simulink model "Coeff_converter_0"  (R2018b)
settings: Solver=VariableStepAuto  StartTime=0.0  StopTime=256  RelTol=1e-3
libraries: xbsIndex_r4 x38
settings Model: Creator=Dima  LastModifiedBy=Dima

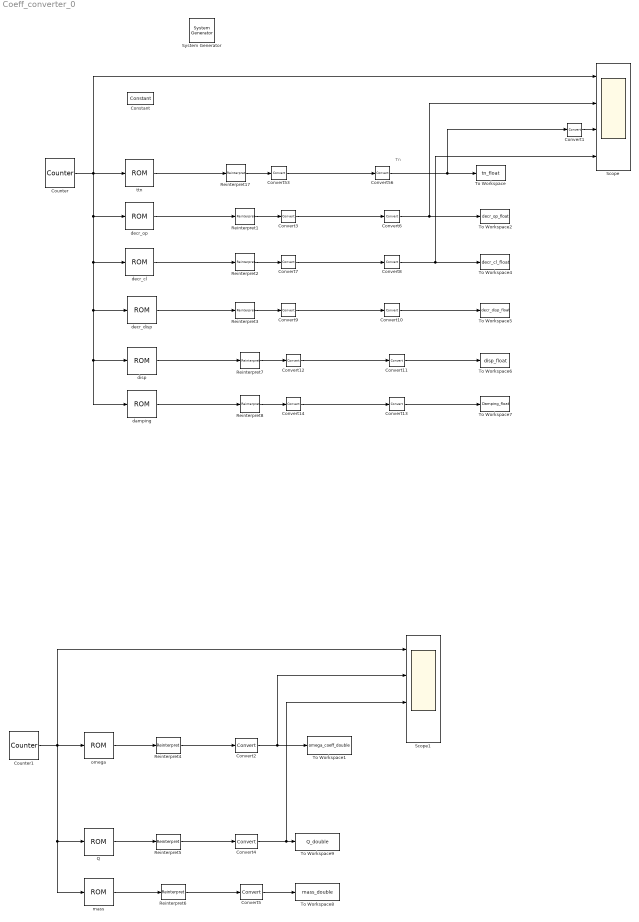
== system Coeff_converter_0 ==
  note: Tn
  " System Generator" : xbsIndex_r4/ System Generator  Tag=genX  xilinxfamily=artix7  part=xc7a35t  speed=-2  package=ftg256  synthesis_tool=Vivado  clock_wrapper=Clock Enables  directory=./netlist  proj_type=Vivado  Synth_file=Vivado Synthesis Defaults  Impl_file=Vivado Implementation Defaults  testbench=off  simulink_period=1  sysclk_period=10  dcm_input_clock_period=10  incr_netlist=off  trim_vbits=Everywhere in SubSystem  dbl_ovrd=According to Block Masks  core_generation=According to Block Masks  run_coregen=off  deprecated_control=off  eval_field=0  block_type=sysgen
  Constant : xbsIndex_r4/Constant  const=18460.73714  gui_display_data_type=Fixed-point  arith_type=Unsigned  n_bits=24  bin_pt=0  preci_type=Single  exp_width=8  frac_width=24  explicit_period=off  period=1  equ=P=C  opselect=C  inp2=PCIN>>17  opr=+  inp1=P  carry=CIN  dbl_ovrd=off  block_type=constant
  Convert{1,6,8,10..11,13,56} (7 alike) : xbsIndex_r4/Convert  gui_display_data_type=Floating-point  arith_type=Floating-point  n_bits=16  bin_pt=14  float_type=Single  exp_bits=8  fraction_bits=24  quantization=Truncate  overflow=Wrap  en=off  latency=0  pipeline=off  dbl_ovrd=off  block_type=convert
  Convert{3,7,9,12,14,53} (6 alike) : xbsIndex_r4/Convert  gui_display_data_type=Fixed-point  arith_type="Signed  (2's comp)"  n_bits=24  bin_pt=23  float_type=Single  exp_bits=8  fraction_bits=24  quantization=Truncate  overflow=Wrap  en=off  latency=0  pipeline=off  dbl_ovrd=off  block_type=convert
  Convert2 : xbsIndex_r4/Convert  gui_display_data_type=Floating-point  arith_type=Floating-point  n_bits=16  bin_pt=14  float_type=Double  exp_bits=8  fraction_bits=24  quantization=Truncate  overflow=Wrap  en=off  latency=0  pipeline=off  dbl_ovrd=off  block_type=convert
  Convert4 : xbsIndex_r4/Convert  gui_display_data_type=Floating-point  arith_type=Floating-point  n_bits=16  bin_pt=14  float_type=Double  exp_bits=8  fraction_bits=24  quantization=Truncate  overflow=Wrap  en=off  latency=0  pipeline=off  dbl_ovrd=off  block_type=convert
  Convert5 : xbsIndex_r4/Convert  gui_display_data_type=Floating-point  arith_type=Floating-point  n_bits=16  bin_pt=14  float_type=Double  exp_bits=8  fraction_bits=24  quantization=Truncate  overflow=Wrap  en=off  latency=0  pipeline=off  dbl_ovrd=off  block_type=convert
  Counter : xbsIndex_r4/Counter  cnt_type=Count Limited  cnt_to=87  operation=Up  start_count=0  cnt_by_val=1  arith_type=Unsigned  n_bits=7  bin_pt=0  load_pin=off  rst=off  en=off  explicit_period=on  period=1  use_behavioral_HDL=off  implementation=Fabric  dbl_ovrd=off  block_type=counter
  Counter1 : xbsIndex_r4/Counter  cnt_type=Free Running  cnt_to=87  operation=Up  start_count=0  cnt_by_val=1  arith_type=Unsigned  n_bits=8  bin_pt=0  load_pin=off  rst=off  en=off  explicit_period=on  period=1  use_behavioral_HDL=off  implementation=Fabric  dbl_ovrd=off  block_type=counter
  Q : xbsIndex_r4/ROM  depth=256  initVector=omega_coef  distributed_mem=Block RAM  rst=off  init_reg=0  en=off  latency=1  gui_display_data_type=Fixed-point  arith_type=Unsigned  n_bits=32  bin_pt=0  preci_type=Single  exp_width=8  frac_width=24  optimize=Area  use_rpm=on  dbl_ovrd=off  block_type=sprom
  Reinterpret{1..3,7..8,17} (6 alike) : xbsIndex_r4/Reinterpret  force_arith_type=off  arith_type="Signed  (2's comp)"  force_bin_pt=on  bin_pt=24  block_type=cast
      settings: block_version=VER_STRING_GOES_HERE
  Reinterpret4 : xbsIndex_r4/Reinterpret  force_arith_type=on  arith_type="Signed  (2's comp)"  force_bin_pt=on  bin_pt=31  block_type=reinterpret
  Reinterpret5 : xbsIndex_r4/Reinterpret  force_arith_type=on  arith_type="Signed  (2's comp)"  force_bin_pt=on  bin_pt=31  block_type=reinterpret
  Reinterpret6 : xbsIndex_r4/Reinterpret  force_arith_type=on  arith_type="Signed  (2's comp)"  force_bin_pt=on  bin_pt=31  block_type=reinterpret
  Scope : Scope  NumInputPorts=4
  Scope1 : Scope  NumInputPorts=4
  To Workspace : ToWorkspace  VariableName=tn_float  SampleTime=-1
  To Workspace1 : ToWorkspace  VariableName=omega_coeff_double  SampleTime=-1
  To Workspace2 : ToWorkspace  VariableName=decr_op_float  SampleTime=-1
  To Workspace4 : ToWorkspace  VariableName=decr_cl_float  SampleTime=-1
  To Workspace5 : ToWorkspace  VariableName=decr_disp_float  SampleTime=-1
  To Workspace6 : ToWorkspace  VariableName=disp_float  SampleTime=-1
  To Workspace7 : ToWorkspace  VariableName=Damping_float  SampleTime=-1
  To Workspace8 : ToWorkspace  VariableName=mass_double  SampleTime=-1
  To Workspace9 : ToWorkspace  VariableName=Q_double  SampleTime=-1
  damping : xbsIndex_r4/ROM  depth=88  initVector=damping  distributed_mem=Block RAM  rst=off  init_reg=0  en=off  latency=1  gui_display_data_type=Fixed-point  arith_type=Unsigned  n_bits=24  bin_pt=0  preci_type=Single  exp_width=8  frac_width=24  optimize=Area  use_rpm=on  dbl_ovrd=off  block_type=sprom
  decr_cl : xbsIndex_r4/ROM  depth=88  initVector=decr_cl  distributed_mem=Block RAM  rst=off  init_reg=0  en=off  latency=1  gui_display_data_type=Fixed-point  arith_type=Unsigned  n_bits=24  bin_pt=0  preci_type=Single  exp_width=8  frac_width=24  optimize=Area  use_rpm=on  dbl_ovrd=off  block_type=sprom
  decr_disp : xbsIndex_r4/ROM  depth=88  initVector=decr_disp  distributed_mem=Block RAM  rst=off  init_reg=0  en=off  latency=1  gui_display_data_type=Fixed-point  arith_type=Unsigned  n_bits=24  bin_pt=0  preci_type=Single  exp_width=8  frac_width=24  optimize=Area  use_rpm=on  dbl_ovrd=off  block_type=sprom
  decr_op : xbsIndex_r4/ROM  depth=88  initVector=decr_op  distributed_mem=Block RAM  rst=off  init_reg=0  en=off  latency=1  gui_display_data_type=Fixed-point  arith_type=Unsigned  n_bits=24  bin_pt=0  preci_type=Single  exp_width=8  frac_width=24  optimize=Area  use_rpm=on  dbl_ovrd=off  block_type=sprom
  disp : xbsIndex_r4/ROM  depth=88  initVector=disp  distributed_mem=Block RAM  rst=off  init_reg=0  en=off  latency=1  gui_display_data_type=Fixed-point  arith_type=Unsigned  n_bits=24  bin_pt=0  preci_type=Single  exp_width=8  frac_width=24  optimize=Area  use_rpm=on  dbl_ovrd=off  block_type=sprom
  mass : xbsIndex_r4/ROM  depth=256  initVector=Mass  distributed_mem=Block RAM  rst=off  init_reg=0  en=off  latency=1  gui_display_data_type=Fixed-point  arith_type=Unsigned  n_bits=32  bin_pt=0  preci_type=Single  exp_width=8  frac_width=24  optimize=Area  use_rpm=on  dbl_ovrd=off  block_type=sprom
  omega : xbsIndex_r4/ROM  depth=256  initVector=omega_coef  distributed_mem=Block RAM  rst=off  init_reg=0  en=off  latency=1  gui_display_data_type=Fixed-point  arith_type=Unsigned  n_bits=32  bin_pt=0  preci_type=Single  exp_width=8  frac_width=24  optimize=Area  use_rpm=on  dbl_ovrd=off  block_type=sprom
  ttn : xbsIndex_r4/ROM  depth=88  initVector=ttn  distributed_mem=Block RAM  rst=off  init_reg=0  en=off  latency=1  gui_display_data_type=Fixed-point  arith_type=Unsigned  n_bits=24  bin_pt=0  preci_type=Single  exp_width=8  frac_width=24  optimize=Area  use_rpm=on  dbl_ovrd=off  block_type=sprom
  wires:
  ttn/1 -> Reinterpret17/1
  Reinterpret17/1 -> Convert53/1
  Convert53/1 -> Convert56/1
  Counter/1 -> Scope/1, decr_op/1, decr_cl/1, decr_disp/1, disp/1, damping/1, ttn/1
  Convert56/1 -> To Workspace/1, Convert1/1
  Convert1/1 -> Scope/3
  Counter1/1 -> Scope1/1, mass/1, Q/1, omega/1
  omega/1 -> Reinterpret4/1
  Reinterpret4/1 -> Convert2/1
  Convert2/1 -> Scope1/2, To Workspace1/1
  decr_op/1 -> Reinterpret1/1
  disp/1 -> Reinterpret7/1
  decr_disp/1 -> Reinterpret3/1
  decr_cl/1 -> Reinterpret2/1
  damping/1 -> Reinterpret8/1
  Reinterpret5/1 -> Convert4/1
  Q/1 -> Reinterpret5/1
  mass/1 -> Reinterpret6/1
  Reinterpret6/1 -> Convert5/1
  Convert5/1 -> To Workspace8/1
  Convert4/1 -> Scope1/3, To Workspace9/1
  ? -> Scope1/4
  Convert6/1 -> Scope/2, To Workspace2/1
  Convert8/1 -> Scope/4, To Workspace4/1
  Convert3/1 -> Convert6/1
  Reinterpret1/1 -> Convert3/1
  Reinterpret2/1 -> Convert7/1
  Convert7/1 -> Convert8/1
  Convert9/1 -> Convert10/1
  Reinterpret3/1 -> Convert9/1
  Reinterpret7/1 -> Convert12/1
  Convert12/1 -> Convert11/1
  Convert14/1 -> Convert13/1
  Reinterpret8/1 -> Convert14/1
  Convert10/1 -> To Workspace5/1
  Convert11/1 -> To Workspace6/1
  Convert13/1 -> To Workspace7/1
